simulink model "Simulink"  (R2020b)
settings: Solver=ode8  StartTime=0.0  StopTime=5  FixedStep=dt  RelTol=1e-3
values from neighbouring files (symbols this model uses):
  K1 = zeros(6,6)    [Main1_Without_Leader.m]    (also in Main2_With_Leader.m)
  L = full(laplacian(G))    [Main1_Without_Leader.m]    (also in Main2_With_Leader.m)
  T = 0.01    [Main1_Without_Leader.m]    (also in Main2_With_Leader.m = 0.0025)
  XY0 = [p1_0';p2_0';p3_0';p4_0';p5_0';p6_0']-ones(6,2)*[3 0;0 2]    [Main1_Without_Leader.m]    (also in Main2_With_Leader.m)
  XYd = [0,0;-1,sqrt(3);1,sqrt(3);1,2+sqrt(3);-1,2+sqrt(3);0,2+2*sqrt(3)]/2    [Main1_Without_Leader.m]    (also in Main2_With_Leader.m)
settings Model: Creator=sokra  LastModifiedBy=sokra

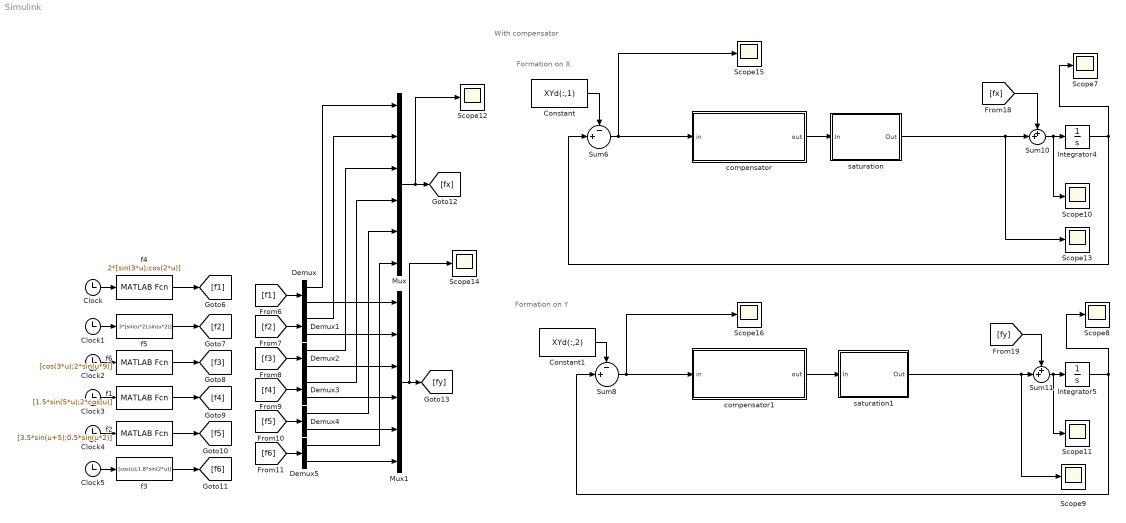
== system Simulink ==
  note: With compensator
  note: Formation on X
  note: Formation on Y
  Clock{,1..5} (6 alike) : Clock
  Constant : Constant  Value=XYd(:,1)
  Constant1 : Constant  Value=XYd(:,2)
  Demux{,1..5} (6 alike) : Demux  Outputs=2
  Integrator4 : Integrator  InitialCondition=XY0(:,1)
  Integrator5 : Integrator  InitialCondition=XY0(:,2)
  Mux : Mux  Inputs=6
  Mux1 : Mux  Inputs=6
  Scope{7..16} (10 alike) : Scope
  Sum10 : Sum  Inputs=++|
  Sum11 : Sum  Inputs=++|
  Sum6 : Sum  Inputs=-+|
  Sum8 : Sum  Inputs=-+|
  compensator : Subsystem  mask{a=1/T^2, b=2/T}
  compensator1 : Subsystem  mask{a=1/T^2, b=2/T}
  f1 : MATLABFcn  MATLABFcn=[1.5*sin(5*u);2*cos(u)]
  f2 : MATLABFcn  MATLABFcn=[3.5*sin(u+5);0.5*sin(u*2)]
  f3 : MATLABFcn  MATLABFcn=[cos(u);1.8*sin(2*u)]
  f4 : MATLABFcn  MATLABFcn=2*[sin(3*u);cos(2*u)]
  f5 : MATLABFcn  MATLABFcn=3*[sin(u*2);sin(u*2)]
  f6 : MATLABFcn  MATLABFcn=[cos(3*u);2*sin(u*9)]
  saturation : Subsystem  mask{u_max=10, sigma=1e6}
  saturation1 : Subsystem  mask{u_max=10, sigma=1e6}
  wires:
  Clock/1 -> f4/1
  Clock1/1 -> f5/1
  Clock2/1 -> f6/1
  Clock3/1 -> f1/1
  Clock4/1 -> f2/1
  Clock5/1 -> f3/1
  Sum6/1 -> compensator/1(in), Scope15/1
  Constant1/1 -> Sum8/1
  Sum11/1 -> Scope11/1, Integrator5/1
  Constant/1 -> Sum6/1
  saturation/1(Out) -> Scope13/1, Sum10/2
  Integrator4/1 -> Scope7/1, Sum6/2
  compensator/1(out) -> saturation/1(In)
  Sum10/1 -> Scope10/1, Integrator4/1
  Integrator5/1 -> Scope8/1, Sum8/2
  [f1] -> Demux/1
  [f2] -> Demux1/1
  [f3] -> Demux2/1
  [f6] -> Demux5/1
  [f5] -> Demux4/1
  [f4] -> Demux3/1
  f5/1 -> [f2]
  f4/1 -> [f1]
  f6/1 -> [f3]
  f1/1 -> [f4]
  f2/1 -> [f5]
  f3/1 -> [f6]
  Demux/1 -> Mux/1
  Demux1/1 -> Mux/2
  Demux2/1 -> Mux/3
  Demux3/1 -> Mux/4
  Demux4/1 -> Mux/5
  Demux5/1 -> Mux/6
  Demux/2 -> Mux1/1
  Demux1/2 -> Mux1/2
  Demux2/2 -> Mux1/3
  Demux3/2 -> Mux1/4
  Demux4/2 -> Mux1/5
  Demux5/2 -> Mux1/6
  Mux/1 -> Scope12/1, [fx]
  Mux1/1 -> Scope14/1, [fy]
  [fy] -> Sum11/1
  [fx] -> Sum10/1
  compensator1/1(out) -> saturation1/1(In)
  saturation1/1(Out) -> Scope9/1, Sum11/2
  Sum8/1 -> compensator1/1(in), Scope16/1

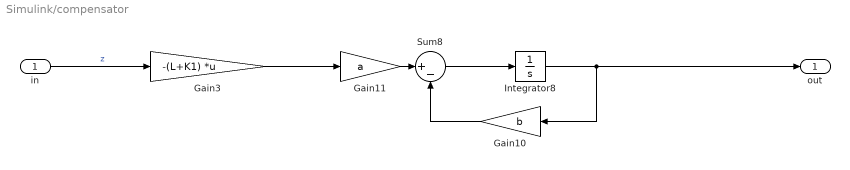
== system Simulink/compensator ==
  in : Inport
  Gain10 : Gain  Gain=b
  Gain11 : Gain  Gain=a
  Gain3 : Gain  Gain=-(L+K1)  Multiplication=Matrix(K*u)
  Integrator8 : Integrator
  Sum8 : Sum  Inputs=|+-
  out : Outport
  wires:
  Gain10/1 -> Sum8/2
  Gain3/1 -> Gain11/1
  Gain11/1 -> Sum8/1
  Integrator8/1 -> Gain10/1, out/1
  Sum8/1 -> Integrator8/1
  in/1 -> Gain3/1  "z"

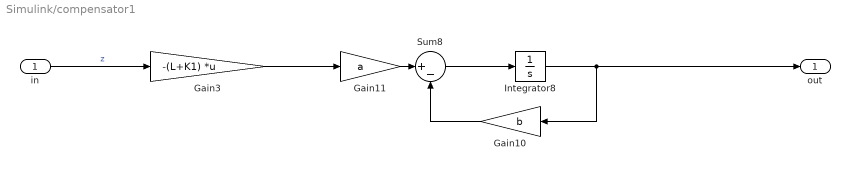
== system Simulink/compensator1 ==
  in : Inport
  Gain10 : Gain  Gain=b
  Gain11 : Gain  Gain=a
  Gain3 : Gain  Gain=-(L+K1)  Multiplication=Matrix(K*u)
  Integrator8 : Integrator
  Sum8 : Sum  Inputs=|+-
  out : Outport
  wires:
  in/1 -> Gain3/1  "z"
  Sum8/1 -> Integrator8/1
  Integrator8/1 -> out/1, Gain10/1
  Gain11/1 -> Sum8/1
  Gain3/1 -> Gain11/1
  Gain10/1 -> Sum8/2

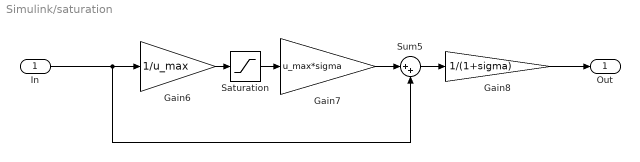
== system Simulink/saturation ==
  In : Inport
  Gain6 : Gain  Gain=1/u_max
  Gain7 : Gain  Gain=u_max*sigma
  Gain8 : Gain  Gain=1/(1+sigma)
  Saturation : Saturate  UpperLimit=1  LowerLimit=-1
  Sum5 : Sum  Inputs=|++
  Out : Outport
  wires:
  Saturation/1 -> Gain7/1
  Gain8/1 -> Out/1
  In/1 -> Sum5/2, Gain6/1
  Gain6/1 -> Saturation/1
  Sum5/1 -> Gain8/1
  Gain7/1 -> Sum5/1

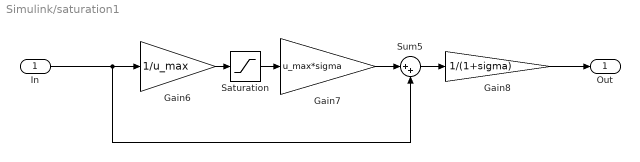
== system Simulink/saturation1 ==
  In : Inport
  Gain6 : Gain  Gain=1/u_max
  Gain7 : Gain  Gain=u_max*sigma
  Gain8 : Gain  Gain=1/(1+sigma)
  Saturation : Saturate  UpperLimit=1  LowerLimit=-1
  Sum5 : Sum  Inputs=|++
  Out : Outport
  wires:
  Gain7/1 -> Sum5/1
  Sum5/1 -> Gain8/1
  Gain6/1 -> Saturation/1
  In/1 -> Gain6/1, Sum5/2
  Gain8/1 -> Out/1
  Saturation/1 -> Gain7/1
